simulink model "minimizer_not_working"  (R2014a)
settings: Solver=ode45  StartTime=0.0  StopTime=10.0  RelTol=1e-3
values from neighbouring files (symbols this model uses):
  I = 1/12*m*((2*ry1)^2 + (2*rx1)^2)    (= 7.53502955357)    [parameters1.m]
  inputBound = [minInput maxInput]    [parameters1.m]
  K = [1000 1000 1000 10 10 1 1]    [parameters1.m]
  m = 46.27    [parameters1.m]
  rx1 = rx01    [Minimizer.m]    (also in parameters1.m = -0.635)
  rx2 = rx02    [Minimizer.m]    (also in parameters1.m = -0.635)
  ry1 = ry01    [Minimizer.m]    (also in parameters1.m = 0.2921)
  ry2 = ry02    [Minimizer.m]    (also in parameters1.m = -0.2921)
undefined symbols (not defined in the file): gain
settings Model: Creator=propagator  LastModifiedBy=propagator
settings OptimizationCC: SimCompilerOptimization=On
settings HardwareCC: ProdBitPerLong=64  ProdBitPerPointer=64  ProdIntDivRoundTo=Zero  ProdEndianess=LittleEndian  ProdWordSize=64  ProdHWDeviceType=Intel->x86-64
settings ModelReferenceCC: EnableParallelModelReferenceBuilds=on
settings RTWCC: BuildConfiguration=Faster Runs  TargetLang=C++
settings GRTTargetCC: MultiInstanceERTCode=on  CodeInterfacePackaging=C++ class

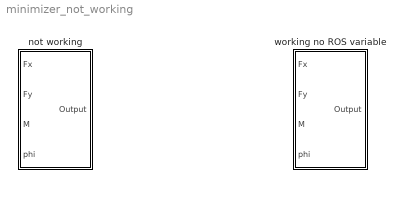
== system minimizer_not_working ==
  not working : Subsystem  mask{rx1=rx1, rx2=rx2, ry1=ry1, ry2=ry2, C=gain, inputBound=inputBound, m=m, I=I}
      mask prompts: C "Performance Gain"; inputBound "Input Bounds"; m "Boat Mass"; I "Boat Inertia"
      mask TypeOptions m: Constant6/Value
      mask TypeOptions I: Constant7/Value
  working no ROS variable : Subsystem  mask{rx1=rx1, rx2=rx2, ry1=ry1, ry2=ry2, C=K, inputBound=inputBound, m=m, I=I}
      mask prompts: C "Performance Gain"; inputBound "Input Bounds"; m "Boat Mass"; I "Boat Inertia"
      mask TypeOptions m: Constant6/Value
      mask TypeOptions I: Constant7/Value

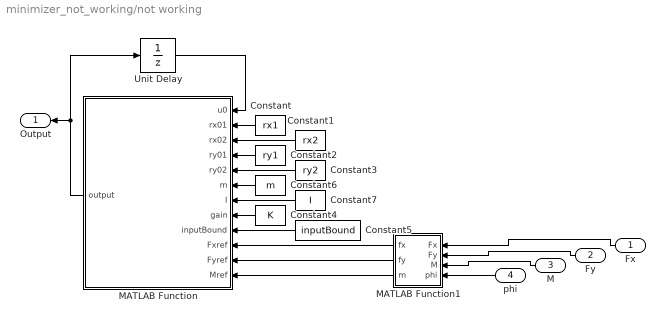
== system minimizer_not_working/not working ==
  Fx : Inport
  Fy : Inport  Port=2
  M : Inport  Port=3
  phi : Inport  Port=4
  Constant : Constant  Value=rx1
  Constant1 : Constant  Value=rx2
  Constant2 : Constant  Value=ry1
  Constant3 : Constant  Value=ry2
  Constant4 : Constant  Value=K
  Constant5 : Constant  Value=inputBound
  Constant6 : Constant  Value=m
  Constant7 : Constant  Value=I
  MATLAB Function : MATLAB Function  TreatAsAtomicUnit=on
  MATLAB Function1 : MATLAB Function  TreatAsAtomicUnit=on
  Unit Delay : UnitDelay  InitialCondition=[0;0;0;0]  SampleTime=-1
  Output : Outport
  wires:
  Constant/1 -> MATLAB Function/2(rx01)
  Constant1/1 -> MATLAB Function/3(rx02)
  Constant2/1 -> MATLAB Function/4(ry01)
  Constant4/1 -> MATLAB Function/8(gain)
  Unit Delay/1 -> MATLAB Function/1(u0)
  MATLAB Function/1(output) -> Unit Delay/1, Output/1
  Constant5/1 -> MATLAB Function/9(inputBound)
  Constant3/1 -> MATLAB Function/5(ry02)
  MATLAB Function1/3(m) -> MATLAB Function/12(Mref)
  MATLAB Function1/2(fy) -> MATLAB Function/11(Fyref)
  MATLAB Function1/1(fx) -> MATLAB Function/10(Fxref)
  Fy/1 -> MATLAB Function1/2(Fy)
  Fx/1 -> MATLAB Function1/1(Fx)
  M/1 -> MATLAB Function1/3(M)
  phi/1 -> MATLAB Function1/4(phi)
  Constant6/1 -> MATLAB Function/6(m)
  Constant7/1 -> MATLAB Function/7(I)

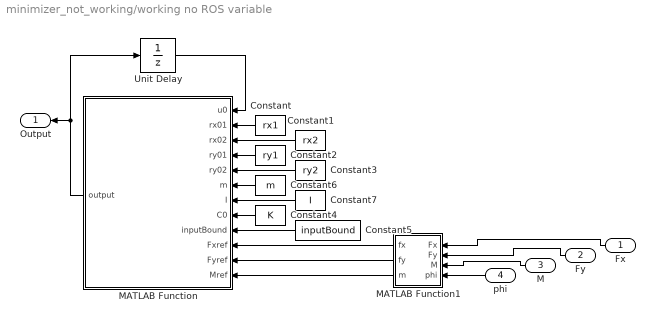
== system minimizer_not_working/working no ROS variable ==
  Fx : Inport
  Fy : Inport  Port=2
  M : Inport  Port=3
  phi : Inport  Port=4
  Constant : Constant  Value=rx1
  Constant1 : Constant  Value=rx2
  Constant2 : Constant  Value=ry1
  Constant3 : Constant  Value=ry2
  Constant4 : Constant  Value=K
  Constant5 : Constant  Value=inputBound
  Constant6 : Constant  Value=m
  Constant7 : Constant  Value=I
  MATLAB Function : MATLAB Function  TreatAsAtomicUnit=on
  MATLAB Function1 : MATLAB Function  TreatAsAtomicUnit=on
  Unit Delay : UnitDelay  InitialCondition=[0;0;0;0]  SampleTime=-1
  Output : Outport
  wires:
  Constant/1 -> MATLAB Function/2(rx01)
  Constant1/1 -> MATLAB Function/3(rx02)
  Constant2/1 -> MATLAB Function/4(ry01)
  Constant4/1 -> MATLAB Function/8(C0)
  Unit Delay/1 -> MATLAB Function/1(u0)
  MATLAB Function/1(output) -> Unit Delay/1, Output/1
  Constant5/1 -> MATLAB Function/9(inputBound)
  Constant3/1 -> MATLAB Function/5(ry02)
  MATLAB Function1/3(m) -> MATLAB Function/12(Mref)
  MATLAB Function1/2(fy) -> MATLAB Function/11(Fyref)
  MATLAB Function1/1(fx) -> MATLAB Function/10(Fxref)
  Fy/1 -> MATLAB Function1/2(Fy)
  Fx/1 -> MATLAB Function1/1(Fx)
  M/1 -> MATLAB Function1/3(M)
  phi/1 -> MATLAB Function1/4(phi)
  Constant6/1 -> MATLAB Function/6(m)
  Constant7/1 -> MATLAB Function/7(I)

== matlab function minimizer_not_working/working no ROS variable/MATLAB Function ==
  data: u0 input; output output; rx01 input; rx02 input; ry01 input; ry02 input; m input; I input; C0 input; inputBound input; Fxref input; Fyref input; Mref input
function output = Minimizer(u0, rx01, rx02, ry01, ry02, m, I, C0, inputBound, Fxref, Fyref, Mref)

rx1 = rx01; rx2 = rx02;
ry1 = ry01; ry2 = ry02;

C = C0;

%Fxref = Fx; Fyref = Fy; Mref  = M;

gridNum = 10;

grid = boundGrid(inputBound, gridNum, rx1,ry1);

u1 = getMinFromGrid(grid, u0, Fxref, Fyref, Mref, rx1, rx2, ry1, ry2, C, m, I);

% u1 = u0;

% %     for k = 1:20
% %         h = getDirection(u1, u0, Fxref, Fyref, Mref, rx1, rx2, ry1, ry2, C);
% %         alpha = getStepSize(u1, u0, h, Fxref, Fyref, Mref, rx1, rx2, ry1, ry2, C);
% %         u1 = u1 + alpha*h;
% %         u1 = checkInputBound(u1,inputBound);
% %     end
    
    output = u1;

end

function output = getMinFromGrid(grid, preinput, Fxref, Fyref, Mref, rx1, rx2, ry1, ry2, C, m, I)

[ii, iii] = size(grid);
v0 = costFunction(grid(1,:), preinput, Fxref, Fyref, Mref, rx1, rx2, ry1, ry2, C, m, I);

output = [grid(1,1);grid(1,2);grid(1,3);grid(1,4)];

for i = 1:ii
    for j = 1:ii
        for k = 1:ii
            for l = 1:ii
                input = [grid(i,1);grid(j,2);grid(k,3);grid(l,4)];
                v1 = costFunction(input,preinput, Fxref, Fyref, Mref, rx1, rx2, ry1, ry2, C, m, I);
                if v0 > v1
                    v0 = v1;
                    output = input;
                else
                end
            end
        end
    end
end

end

function output = checkInputBound(input,inputBound)
k = [0;0;0;0];
    for i = 1:length(input)
        k(i) = sat(input(i),inputBound(i,:));
    end
    output = k;
end

function output = boundGrid(inputBound, gridNum, rx1,ry1)

p = gridNum;

current_port_servo_angle =    [0.2664;0.1837;0.1010;0.0184;-0.0643;-0.1470;-0.2296;-0.3123;-0.3950;-0.4777;...
-0.5603;-0.6430;-0.7257;-0.8084;-0.8910;-0.9737;-1.0564;-1.1054;-1.1391;-1.2217]*180/pi;                      %linspace(inputBound(1,1),inputBound(1,2),p)';
current_port_thruster_force =        [39.25;30;20;10;5;0;-5;-10;-15;-23.65;zeros(10,1)];                                                             %linspace(inputBound(2,1),inputBound(2,2),p)';
current_starboard_servo_angle =    [0.2664;0.1837;0.1010;0.0184;-0.0643;-0.1470;-0.2296;-0.3123;-0.3950;-0.4777;...
-0.5603;-0.6430;-0.7257;-0.8084;-0.8910;-0.9737;-1.0564;-1.1054;-1.1391;-1.2217]*-180/pi;                      %linspace(inputBound(3,1),inputBound(3,2),p)';
current_starboard_thruster_force =        [39.25;30;20;10;5;0;-5;-10;-15;-23.65;zeros(10,1)];                                                            %linspace(inputBound(4,1),inputBound(4,2),p)';

%i = atan(rx1/ry1)*180/pi;

output = [current_port_servo_angle, current_port_thruster_force, current_starboard_servo_angle, current_starboard_thruster_force];%;...
%           inputBound(1,1),  0,      inputBound(3,1),  0;...
%              0,    100,    0,    100;...%];
%              0,   -100,    0,   -100]; %...
%             i,    0,    i,    0];

% p = gridNum;
% 
% theta1 =    linspace(inputBound(1,1),inputBound(1,2),p)';
% f1 =        linspace(inputBound(2,1),inputBound(2,2),p)';
% theta2 =    linspace(inputBound(3,1),inputBound(3,2),p)';
% f2 =        linspace(inputBound(4,1),inputBound(4,2),p)';
% 
% %i = atan(rx1/ry1)*180/pi;
% 
% output = [theta1, f1, theta2, f2;...
%           inputBound(1,1),  0,      inputBound(3,1),  0;...
%              0,    100,    0,    100;...%];
%              0,   -100,    0,   -100]; %...
% %             i,    0,    i,    0];

end

function output = sat(input, bound)

    if input < bound(1)
        output = bound(1);
    elseif input > bound(2)
        output = bound(2);
    else
        output = input;
    end

end

function output = getStepSize(input, preinput, h, Fxref, Fyref, Mref, rx1, rx2, ry1, ry2, C, m, I)

    alpha = .001;
    
    u0 = input;
    u1 = input + alpha*h;
    
    v0 = costFunction( u0, preinput, Fxref, Fyref, Mref, rx1, rx2, ry1, ry2, C, m, I );
    v1 = costFunction( u1, preinput, Fxref, Fyref, Mref, rx1, rx2, ry1, ry2, C, m, I);

    while v1 <= v0 && v1 ~= 0
        alpha = alpha + .001;
        u1 = input + alpha*h;
        v0 = v1;
        v1 = costFunction( u1, preinput, Fxref, Fyref, Mref, rx1, rx2, ry1, ry2, C, m, I );
    end
    
    v0 = v1;
    alpha = .0015;

    while v1 <= v0  && v1 ~= 0
        alpha = alpha - 0.0001;
        u1 = input + alpha*h;
        v0 = v1;
        v1 = costFunction( u1, preinput, Fxref, Fyref, Mref, rx1, rx2, ry1, ry2, C, m, I );
    end


    output = alpha;

end

function output = costFunction(input, preinput, Fxref, Fyref, Mref, rx1, rx2, ry1, ry2, C, m, I)

    theta1  = input(1);
    f1      = input(2);
    theta2  = input(3);
    f2      = input(4);
    
    pretheta1   = preinput(1);
    pretheta2   = preinput(3);

    Fx = f1*cosd(theta1) + f2*cosd(theta2);
    Fy = f1*sind(theta1) + f2*sind(theta2);
    M = -rx1*f1*sind(theta1) + ry1*f1*cosd(theta1) - rx2*f2*sind(theta2)...
        + ry2*f2*cosd(theta2);

    output = C(1)*(Fx-Fxref)^2 +...
        C(2)*(Fy-Fyref)^2 +...
        C(3)*(M-Mref)^2  +...
        C(4)*f1^2 +...
        C(5)*f2^2 +...
        C(6)*(theta1 - pretheta1)^2 +...
        C(7)*(theta2 - pretheta2)^2;% +...
%         C(5)*theta1^2 +...
%         C(5)*theta2^2;

end

function output = getDirection(input, preinput, Fxref, Fyref, Mref, rx1, rx2, ry1, ry2, C, m, I)

hsd = SteepestDescent(input, preinput, Fxref, Fyref, Mref, rx1, rx2, ry1, ry2, C, m, I);

output = zeros(4,1);

    for i = 1:length(hsd)
        output(i) = hsd(i);
    end
    
end

function output = SteepestDescent(input, preinput, Fxref, Fyref, Mref, rx1, rx2, ry1, ry2, C, m, I)

theta1  = input(1);
f1      = input(2);
theta2  = input(3);
f2      = input(4);

pretheta1   = preinput(1);
pretheta2   = preinput(3);

dVdtheta1 = C(3)*(f1*ry1*cosd(theta1)...
    - f1*rx1*sind(theta1))*(f1*rx1*cosd(theta1)...
    - Mref + f2*rx2*cosd(theta2) + f1*ry1*sin(theta1)...
    + f2*ry2*sind(theta2)) - C(6)*(pretheta1 - theta1)...
    - C(2)*f1*sind(theta1)*(f1*cosd(theta1) - Fyref + f2*cosd(theta2))...
    + C(1)*f1*cosd(theta1)*(Fxref + f1*sind(theta1) + f2*sind(theta2));

dVdf1 = C(4)*f1 + C(1)*sind(theta1)*(Fxref + f1*sin(theta1)...
    + f2*sind(theta2)) + C(2)*cosd(theta1)*(f1*cosd(theta1) - Fyref...
    + f2*cosd(theta2)) + C(3)*(rx1*cosd(theta1)...
    + ry1*sind(theta1))*(f1*rx1*cosd(theta1) - Mref + f2*rx2*cosd(theta2)...
    + f1*ry1*sind(theta1) + f2*ry2*sind(theta2));

dVdtheta2 = C(3)*(f2*ry2*cosd(theta2)...
    - f2*rx2*sind(theta2))*(f1*rx1*cosd(theta1)...
    - Mref + f2*rx2*cosd(theta2) + f1*ry1*sind(theta1)...
    + f2*ry2*sind(theta2)) - C(7)*(pretheta2 - theta2)...
    - C(2)*f2*sind(theta2)*(f1*cosd(theta1) - Fyref + f2*cosd(theta2))...
    + C(1)*f2*cosd(theta2)*(Fxref + f1*sind(theta1) + f2*sind(theta2));

dVdf2 = C(5)*f2 + C(1)*sind(theta2)*(Fxref + f1*sind(theta1)...
    + f2*sind(theta2)) + C(2)*cosd(theta2)*(f1*cosd(theta1) - Fyref...
    + f2*cosd(theta2)) + C(3)*(rx2*cosd(theta2)...
    + ry2*sind(theta2))*(f1*rx1*cosd(theta1) - Mref + f2*rx2*cosd(theta2)...
    + f1*ry1*sind(theta1) + f2*ry2*sind(theta2));
 
output = -[dVdtheta1; dVdf1; dVdtheta2; dVdf2];

end

== matlab function minimizer_not_working/working no ROS variable/MATLAB Function1 ==
  data: Fx input; fx output; Fy input; M input; fy output; m output; phi input
function [fx,fy,m] = fcn(Fx,Fy,M, phi)
%#codegen

R = [cosd(phi) -sind(phi) 0;...
        sind(phi)  cosd(phi) 0;...
        0           0       1];
    
    FxyM = R'*[Fx;Fy;M];
    
    fx = FxyM(1);
    fy = FxyM(2);
    m = FxyM(3);
    
end

== matlab function minimizer_not_working/not working/MATLAB Function ==
  data: u0 input; output output; rx01 input; rx02 input; ry01 input; ry02 input; m input; I input; gain input; inputBound input; Fxref input; Fyref input; Mref input
function output = Minimizer(u0, rx01, rx02, ry01, ry02, m, I, gain, inputBound, Fxref, Fyref, Mref)

rx1 = rx01; rx2 = rx02;
ry1 = ry01; ry2 = ry02;



%Fxref = Fx; Fyref = Fy; Mref  = M;

gridNum = 10;

grid = boundGrid(inputBound, gridNum, rx1,ry1);

u1 = getMinFromGrid(grid, u0, Fxref, Fyref, Mref, rx1, rx2, ry1, ry2, gain, m, I);

% u1 = u0;

% %     for k = 1:20
% %         h = getDirection(u1, u0, Fxref, Fyref, Mref, rx1, rx2, ry1, ry2, C);
% %         alpha = getStepSize(u1, u0, h, Fxref, Fyref, Mref, rx1, rx2, ry1, ry2, C);
% %         u1 = u1 + alpha*h;
% %         u1 = checkInputBound(u1,inputBound);
% %     end

u1(1) = u1(1)*pi/180;
u1(3) = u1(3)*pi/180;
    
    output = u1;

end

function output = getMinFromGrid(grid, preinput, Fxref, Fyref, Mref, rx1, rx2, ry1, ry2, gain, m, I)

[ii, iii] = size(grid);
v0 = 1*costFunction(grid(1,:), preinput, Fxref, Fyref, Mref, rx1, rx2, ry1, ry2, gain, m, I);

output = [grid(1,1);grid(1,2);grid(1,3);grid(1,4)];

for i = 1:ii
    for j = 1:ii
        for k = 1:ii
            for l = 1:ii
                input = [grid(i,1);grid(j,2);grid(k,3);grid(l,4)];
                v1 = 1*costFunction(input,preinput, Fxref, Fyref, Mref, rx1, rx2, ry1, ry2, gain, m, I);
                if v0 > v1
                    v0 = v1;
                    output = input;
                else
                end
            end
        end
    end
end

end

function output = checkInputBound(input,inputBound)
k = [0;0;0;0];
    for i = 1:length(input)
        k(i) = sat(input(i),inputBound(i,:));
    end
    output = k;
end

function output = boundGrid(inputBound, gridNum, rx1,ry1)

p = gridNum;

current_port_servo_angle =    [0.2664;0.1837;0.1010;0.0184;-0.0643;-0.1470;-0.2296;-0.3123;-0.3950;-0.4777;...
-0.5603;-0.6430;-0.7257;-0.8084;-0.8910;-0.9737;-1.0564;-1.1054;-1.1391;-1.2217]*180/pi;                      %linspace(inputBound(1,1),inputBound(1,2),p)';
current_port_thruster_force =        [39.25;30;20;10;5;0;-5;-10;-15;-23.65;zeros(10,1)];                                                             %linspace(inputBound(2,1),inputBound(2,2),p)';
current_starboard_servo_angle =    [0.2664;0.1837;0.1010;0.0184;-0.0643;-0.1470;-0.2296;-0.3123;-0.3950;-0.4777;...
-0.5603;-0.6430;-0.7257;-0.8084;-0.8910;-0.9737;-1.0564;-1.1054;-1.1391;-1.2217]*-180/pi;                      %linspace(inputBound(3,1),inputBound(3,2),p)';
current_starboard_thruster_force =        [39.25;30;20;10;5;0;-5;-10;-15;-23.65;zeros(10,1)];                                                            %linspace(inputBound(4,1),inputBound(4,2),p)';

%i = atan(rx1/ry1)*180/pi;

output = [current_port_servo_angle, current_port_thruster_force, current_starboard_servo_angle, current_starboard_thruster_force];%;...
%           inputBound(1,1),  0,      inputBound(3,1),  0;...
%              0,    100,    0,    100;...%];
%              0,   -100,    0,   -100]; %...
%             i,    0,    i,    0];

end

function output = sat(input, bound)

    if input < bound(1)
        output = bound(1);
    elseif input > bound(2)
        output = bound(2);
    else
        output = input;
    end

end

% function output = getStepSize(input, preinput, h, Fxref, Fyref, Mref, rx1, rx2, ry1, ry2, gain, m, I)
% 
%     alpha = .001;
%     
%     u0 = input;
%     u1 = input + alpha*h;
%     
%     v0 = costFunction( u0, preinput, Fxref, Fyref, Mref, rx1, rx2, ry1, ry2, gain, m, I );
%     v1 = costFunction( u1, preinput, Fxref, Fyref, Mref, rx1, rx2, ry1, ry2, gain, m, I);
% 
%     while v1 <= v0 && v1 ~= 0
%         alpha = alpha + .001;
%         u1 = input + alpha*h;
%         v0 = v1;
%         v1 = costFunction( u1, preinput, Fxref, Fyref, Mref, rx1, rx2, ry1, ry2, gain, m, I );
%     end
%     
%     v0 = v1;
%     alpha = .0015;
% 
%     while v1 <= v0  && v1 ~= 0
%         alpha = alpha - 0.0001;
%         u1 = input + alpha*h;
%         v0 = v1;
%         v1 = costFunction( u1, preinput, Fxref, Fyref, Mref, rx1, rx2, ry1, ry2, gain, m, I );
%     end
% 
% 
%     output = alpha;
% 
% end

function output = costFunction(input, preinput, Fxref, Fyref, Mref, port_servo_x_offset, starboard_servo_x_offset, port_servo_y_offset, starboard_servo_y_offset, gain, m, I)

    port_servo_angle  = input(1);
    port_thruster_force      = input(2);
    starboard_servo_angle  = input(3);
    starboard_thruster_force      = input(4);
    
    current_port_servo_angle   = preinput(1);
    current_starboard_servo_angle   = preinput(3);

    Fx = (port_thruster_force*cosd(port_servo_angle) + starboard_thruster_force*cosd(starboard_servo_angle));
    Fy = (port_thruster_force*sind(port_servo_angle) + starboard_thruster_force*sind(starboard_servo_angle));
    M = (-port_servo_x_offset*port_thruster_force*sind(port_servo_angle) + port_servo_y_offset*port_thruster_force*cosd(port_servo_angle)... 
        - starboard_servo_x_offset*starboard_thruster_force*sind(starboard_servo_angle) + starboard_servo_y_offset*starboard_thruster_force*cosd(starboard_servo_angle));

    output = gain.error_force_x/2               * (Fx-Fxref)^2 +...
        gain.error_force_y/2                    * (Fy-Fyref)^2 +...
        gain.error_moment_z/2                   * (M-Mref)^2  +...
        gain.thruster_force/2                   * port_thruster_force^2 +...
        gain.thruster_force/2                   * starboard_thruster_force^2 +...
        gain.deviation_equilibrum_servo_angle/2 * port_servo_angle^2 +...
        gain.deviation_equilibrum_servo_angle/2 * starboard_servo_angle^2 +...
        gain.deviation_changeof_servo_angle/2   * (port_servo_angle - current_port_servo_angle)^2 +...
        gain.deviation_changeof_servo_angle/2   * (starboard_servo_angle - current_starboard_servo_angle)^2;

end

% function output = getDirection(input, preinput, Fxref, Fyref, Mref, rx1, rx2, ry1, ry2, gain, m, I)
% 
% hsd = SteepestDescent(input, preinput, Fxref, Fyref, Mref, rx1, rx2, ry1, ry2, gain, m, I);
% 
% output = zeros(4,1);
% 
%     for i = 1:length(hsd)
%         output(i) = hsd(i);
%     end
%     
% end

% function output = SteepestDescent(input, preinput, Fxref, Fyref, Mref, rx1, rx2, ry1, ry2, gain, m, I)
% 
% theta1  = input(1);
% f1      = input(2);
% theta2  = input(3);
% f2      = input(4);
% 
% pretheta1   = preinput(1);
% pretheta2   = preinput(3);
% 
% dVdtheta1 = C(3)*(f1*ry1*cosd(theta1)...
%     - f1*rx1*sind(theta1))*(f1*rx1*cosd(theta1)...
%     - Mref + f2*rx2*cosd(theta2) + f1*ry1*sin(theta1)...
%     + f2*ry2*sind(theta2)) - C(6)*(pretheta1 - theta1)...
%     - C(2)*f1*sind(theta1)*(f1*cosd(theta1) - Fyref + f2*cosd(theta2))...
%     + C(1)*f1*cosd(theta1)*(Fxref + f1*sind(theta1) + f2*sind(theta2));
% 
% dVdf1 = C(4)*f1 + C(1)*sind(theta1)*(Fxref + f1*sin(theta1)...
%     + f2*sind(theta2)) + C(2)*cosd(theta1)*(f1*cosd(theta1) - Fyref...
%     + f2*cosd(theta2)) + C(3)*(rx1*cosd(theta1)...
%     + ry1*sind(theta1))*(f1*rx1*cosd(theta1) - Mref + f2*rx2*cosd(theta2)...
%     + f1*ry1*sind(theta1) + f2*ry2*sind(theta2));
% 
% dVdtheta2 = C(3)*(f2*ry2*cosd(theta2)...
%     - f2*rx2*sind(theta2))*(f1*rx1*cosd(theta1)...
%     - Mref + f2*rx2*cosd(theta2) + f1*ry1*sind(theta1)...
%     + f2*ry2*sind(theta2)) - C(7)*(pretheta2 - theta2)...
%     - C(2)*f2*sind(theta2)*(f1*cosd(theta1) - Fyref + f2*cosd(theta2))...
%     + C(1)*f2*cosd(theta2)*(Fxref + f1*sind(theta1) + f2*sind(theta2));
% 
% dVdf2 = C(5)*f2 + C(1)*sind(theta2)*(Fxref + f1*sind(theta1)...
%     + f2*sind(theta2)) + C(2)*cosd(theta2)*(f1*cosd(theta1) - Fyref...
%     + f2*cosd(theta2)) + C(3)*(rx2*cosd(theta2)...
%     + ry2*sind(theta2))*(f1*rx1*cosd(theta1) - Mref + f2*rx2*cosd(theta2)...
%     + f1*ry1*sind(theta1) + f2*ry2*sind(theta2));
%  
% output = -[dVdtheta1; dVdf1; dVdtheta2; dVdf2];
% 
% end

== matlab function minimizer_not_working/not working/MATLAB Function1 ==
  data: Fx input; fx output; Fy input; M input; fy output; m output; phi input
function [fx,fy,m] = fcn(Fx,Fy,M, phi)
%#codegen

R = [cosd(phi) -sind(phi) 0;...
        sind(phi)  cosd(phi) 0;...
        0           0       1];
    
    FxyM = R'*[Fx;Fy;M];
    
    fx = FxyM(1);
    fy = FxyM(2);
    m = FxyM(3);
    
end
